simulink model "Comau_robot_dig_test"  (R2024b)
settings: Solver=FixedStepAuto  StartTime=0.0  StopTime=inf  FixedStep=Ts  RelTol=1e-3
model workspace (MATLAB code in the model file):
  other statements: smiDataRobot.RigidTransform(16).translation = [0.0 0.0 0.0];; smiDataRobot.RigidTransform(16).angle = 0.0;; smiDataRobot.RigidTransform(16).axis = [0.0 0.0 0.0];; smiDataRobot.RigidTransform(16).ID = "";; smiDataRobot.RigidTransform(1).translation = [0 331 0];  % mm; smiDataRobot.RigidTransform(1).angle = 0;  % rad; smiDataRobot.RigidTransform(1).axis = [0 0 0];; smiDataRobot.RigidTransform(1).ID = "AssemblyGround[SMART-5 NJ-110-3.0 (3D-STEP).STEP-1:SMART-5 NJ-110-3.0_p02.STEP-1]";; smiDataRobot.RigidTransform(2).translation = [-450 2240 0];  % mm; smiDataRobot.RigidTransform(2).angle = 0;  % rad; smiDataRobot.RigidTransform(2).axis = [0 0 0];; smiDataRobot.RigidTransform(2).ID = "AssemblyGround[SMART-5 NJ-110-3.0 (3D-STEP).STEP-1:SMART-5 NJ-110-3.0_p05.STEP-1]"; ... (+161)
values from neighbouring files (symbols this model uses):
  L2 = 830e-3    (= 0.83)    [Robot_parameters.m]
  L3 = 1160e-3    (= 1.16)    [Robot_parameters.m]
  L4 = 250e-3    (= 0.25)    [Robot_parameters.m]
undefined symbols (not defined in the file or in its folder): M, SList, smiDataRobot, thetaList0, X, Y, Z
libraries: sm_lib x78, nesl_utility x18, slrealtimeutilitieslib x2, slrealtimeiplib x2
(part 4 of 4)

== matlab function Comau_robot_dig_test/IK_solver/inverseKinematics ==
  data: p input; thetaList output size=[5, 1]; p_vel input; thetaList0 input; M input; SList input; thetaListDot output size=[5, 1]; success output size=1
function [thetaList, thetaListDot, success] = inverseKinematics( ...
    p, p_vel, thetaList0, M, SList)


T = [1 0 0 p(1);
     0 1 0 p(2);
     0 0 1 p(3);
     0 0 0 1];

[thetaOut, successOut] = IKinSpace(SList, M, T, thetaList0, 0.00001, 0.0000001);


% Assign them to the pre-allocated outputs
thetaList    = thetaOut;
success      = successOut;

%Exploiting linear relationship between q3 and q2 to obtain actual angle of
%of actuated joint
% q3_closure = thetaList(3) - thetaList(2);
% thetaList_closure= [thetaList(1); thetaList(2); q3_closure; thetaList(4); thetaList(5)];


Js = JacobianSpace(SList,thetaList);

%pseudo inverse jacobian
Js_pinv = pinv(Js);
xyzDot = [0;
         0;
         0;
         p_vel(1);
         p_vel(2);
         p_vel(3)
         ];

thetaListDot = Js_pinv*xyzDot;

end
